simulink model "AccelPdl"  (R2023a)
settings: Solver=ode3  StartTime=0.0  StopTime=33  FixedStep=0.001  RelTol=1e-3
values from neighbouring files (symbols this model uses):
  TqCmdEPA_Forward_Final = 434.3391262014984 436.91867797860527 439.498229755712 442.07778153281885 444.65733330992566 447.42381495044009 450.91373414617271 454.40365334190523 457.89357253763791 461.38349173337048 463.56484227432378 463.86833033972778 464.17181840513183 464.47530647053583 464.77879453593988 464.89533286466883 464.89533286466883 464.89533286466883 464.89533286466883 464.89533286466883 464.64606655078757 464.    [BeginnerDevModel_Dictionary.sldd]    (also in EPATorqueOutputs.mat = [434.339126201 436.918677979 439.498229756 442.077781533 444; TqCommandGenerator.m = transpose(TqCmd_Array_Reshaped))
  TqCmdEPA_Reverse_Final = -124.07811446556342 -124.07811446556342 -124.07811446556342 -124.07811446556342 -124.0781144658778 -124.07811447343717 -124.07811448099652 -124.07811448855587 -124.07811449548642 -124.07811449548642 -124.07811449548642 -124.07811449548642 -124.07811449548642 -124.07811449548642 -124.07811449548642 -124.07001588912377 -124.01236684976388 -123.95471781040399 -123.89706877104413 -123.83941973168425 -    [BeginnerDevModel_Dictionary.sldd]    (also in EPATorqueOutputs.mat = [-124.078114466 -124.078114466 -124.078114466 -124.078114466; TqCommandGenerator.m = transpose(TqCmd_Array_Reshaped))
settings Model: DataDictionary=BeginnerDevModel_Dictionary.sldd  Creator=edward9  LastModifiedBy=edward9

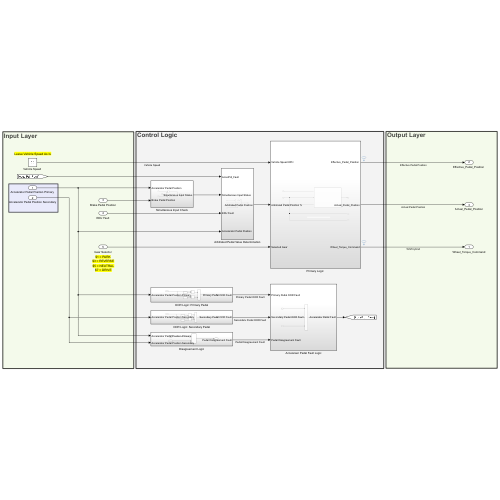
[thumbnail: Simulink's stored preview of the top-level diagram]
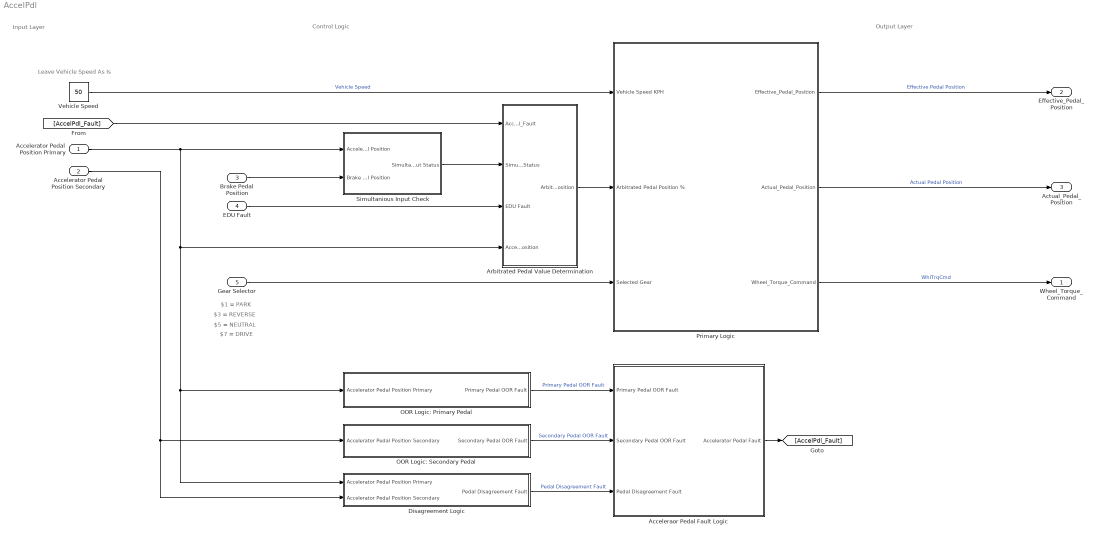
== system AccelPdl ==
  note: $7 = DRIVE
  note: $5 = NEUTRAL
  note: $3 = REVERSE
  note: Control Logic
  note: Input Layer
  note: Output Layer
  note: $1 = PARK
  note: Leave Vehicle Speed As Is
  "Accelerator Pedal Position Primary " : Inport  OutDataTypeStr=double
  Accelerator Pedal Position Secondary : Inport  Port=2  OutDataTypeStr=double
  Brake Pedal Position : Inport  Port=3  OutDataTypeStr=double
  EDU Fault : Inport  Port=4
  Gear Selector : Inport  Port=5  OutDataTypeStr=double
  Acceleraor Pedal Fault Logic : Subsystem
  Arbitrated Pedal Value Determination : Subsystem
  Disagreement Logic : Subsystem
  OOR Logic: Primary Pedal : Subsystem
  OOR Logic: Secondary Pedal : Subsystem
  "Primary Logic " : Subsystem
  Simultanious Input Check : Subsystem
  "Vehicle Speed " : Constant  Value=50
  Wheel_Torque_Command : Outport
  "Effective_Pedal_Position " : Outport  Port=2
  Actual_Pedal_Position : Outport  Port=3
  wires:
  Acceleraor Pedal Fault Logic/1(Accelerator Pedal Fault) -> [AccelPdl_Fault]
  "Vehicle Speed "/1 -> "Primary Logic "/1(Vehicle Speed KPH)  "Vehicle Speed"
  "Primary Logic "/1("Effective_Pedal_Position ") -> "Effective_Pedal_Position "/1  "Effective Pedal Position"
  "Primary Logic "/2(Actual_Pedal_Position) -> Actual_Pedal_Position/1  "Actual Pedal Position"
  Gear Selector/1 -> "Primary Logic "/3(Selected Gear)
  Arbitrated Pedal Value Determination/1(Arbitrated Pedal Position) -> "Primary Logic "/2("Arbitrated Pedal Position % ")
  "Primary Logic "/3(Wheel_Torque_Command) -> Wheel_Torque_Command/1  "WhlTrqCmd"
  Brake Pedal Position/1 -> Simultanious Input Check/2(Brake Pedal Position)
  [AccelPdl_Fault] -> Arbitrated Pedal Value Determination/1(AccelPdl_Fault)
  Simultanious Input Check/1(Simultanious Input Status) -> Arbitrated Pedal Value Determination/2(Simultanious Input Status)
  EDU Fault/1 -> Arbitrated Pedal Value Determination/3(EDU Fault)
  OOR Logic: Secondary Pedal/1(Secondary Pedal OOR Fault) -> Acceleraor Pedal Fault Logic/2(Secondary Pedal OOR Fault)  "Secondary Pedal OOR Fault"
  Disagreement Logic/1(Pedal Disagreement Fault) -> Acceleraor Pedal Fault Logic/3(Pedal Disagreement Fault)  "Pedal Disagreement Fault"
  OOR Logic: Primary Pedal/1(Primary Pedal OOR Fault) -> Acceleraor Pedal Fault Logic/1(Primary Pedal OOR Fault)  "Primary Pedal OOR Fault"
  "Accelerator Pedal Position Primary "/1 -> Simultanious Input Check/1("Accelerator Pedal Position "), Disagreement Logic/1(Accelerator Pedal Position Primary), OOR Logic: Primary Pedal/1(Accelerator Pedal Position Primary), Arbitrated Pedal Value Determination/4(Accelerator Pedal Position)
  Accelerator Pedal Position Secondary/1 -> Disagreement Logic/2(Accelerator Pedal Position Secondary), OOR Logic: Secondary Pedal/1(Accelerator Pedal Position Secondary)

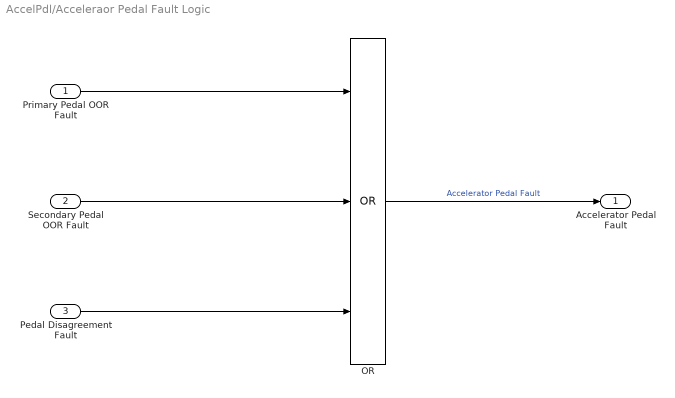
== system AccelPdl/Acceleraor Pedal Fault Logic ==
  Primary Pedal OOR Fault : Inport
  Secondary Pedal OOR Fault : Inport  Port=2
  Pedal Disagreement Fault : Inport  Port=3
  OR : Logic  Operator=OR  Inputs=3  AllPortsSameDT=off  OutDataTypeStr=boolean
  Accelerator Pedal Fault : Outport
  wires:
  Pedal Disagreement Fault/1 -> OR/3
  Secondary Pedal OOR Fault/1 -> OR/2
  Primary Pedal OOR Fault/1 -> OR/1
  OR/1 -> Accelerator Pedal Fault/1  "Accelerator Pedal Fault"

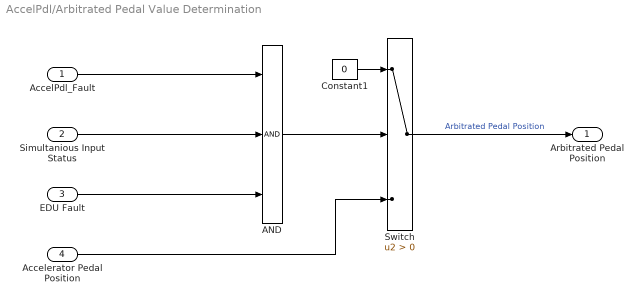
== system AccelPdl/Arbitrated Pedal Value Determination ==
  AccelPdl_Fault : Inport
  Simultanious Input Status : Inport  Port=2
  EDU Fault : Inport  Port=3
  Accelerator Pedal Position : Inport  Port=4
  AND : Logic  Inputs=3  AllPortsSameDT=off  OutDataTypeStr=boolean
  Constant1 : Constant  Value=0
  Switch : Switch  Criteria=u2 > Threshold  SaturateOnIntegerOverflow=off  InputSameDT=off
  Arbitrated Pedal Position : Outport
  wires:
  AccelPdl_Fault/1 -> AND/1
  Accelerator Pedal Position/1 -> Switch/3
  Simultanious Input Status/1 -> AND/2
  AND/1 -> Switch/2
  EDU Fault/1 -> AND/3
  Constant1/1 -> Switch/1
  Switch/1 -> Arbitrated Pedal Position/1  "Arbitrated Pedal Position"

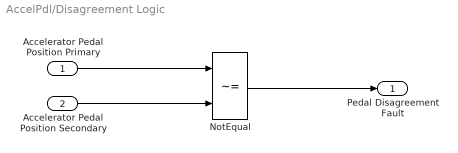
== system AccelPdl/Disagreement Logic ==
  Accelerator Pedal Position Primary : Inport
  Accelerator Pedal Position Secondary : Inport  Port=2
  NotEqual : RelationalOperator  Operator=~=  OutDataTypeStr=boolean  RndMeth=Simplest  InputSameDT=off
  Pedal Disagreement Fault : Outport
  wires:
  NotEqual/1 -> Pedal Disagreement Fault/1
  Accelerator Pedal Position Primary/1 -> NotEqual/1
  Accelerator Pedal Position Secondary/1 -> NotEqual/2

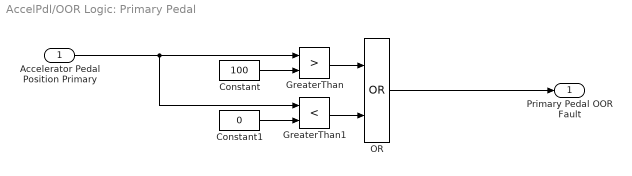
== system AccelPdl/OOR Logic: Primary Pedal ==
  Accelerator Pedal Position Primary : Inport
  Constant : Constant  Value=100
  Constant1 : Constant  Value=0
  GreaterThan : RelationalOperator  Operator=>  OutDataTypeStr=boolean  RndMeth=Simplest  InputSameDT=off
  GreaterThan1 : RelationalOperator  Operator=<  OutDataTypeStr=boolean  RndMeth=Simplest  InputSameDT=off
  OR : Logic  Operator=OR  AllPortsSameDT=off  OutDataTypeStr=boolean
  Primary Pedal OOR Fault : Outport
  wires:
  OR/1 -> Primary Pedal OOR Fault/1
  Constant1/1 -> GreaterThan1/2
  GreaterThan/1 -> OR/1
  GreaterThan1/1 -> OR/2
  Constant/1 -> GreaterThan/2
  Accelerator Pedal Position Primary/1 -> GreaterThan1/1, GreaterThan/1

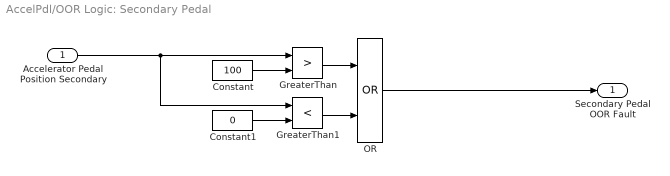
== system AccelPdl/OOR Logic: Secondary Pedal ==
  Accelerator Pedal Position Secondary : Inport
  Constant : Constant  Value=100
  Constant1 : Constant  Value=0
  GreaterThan : RelationalOperator  Operator=>  OutDataTypeStr=boolean  RndMeth=Simplest  InputSameDT=off
  GreaterThan1 : RelationalOperator  Operator=<  OutDataTypeStr=boolean  RndMeth=Simplest  InputSameDT=off
  OR : Logic  Operator=OR  AllPortsSameDT=off  OutDataTypeStr=boolean
  Secondary Pedal OOR Fault : Outport
  wires:
  OR/1 -> Secondary Pedal OOR Fault/1
  Constant1/1 -> GreaterThan1/2
  GreaterThan/1 -> OR/1
  GreaterThan1/1 -> OR/2
  Constant/1 -> GreaterThan/2
  Accelerator Pedal Position Secondary/1 -> GreaterThan1/1, GreaterThan/1

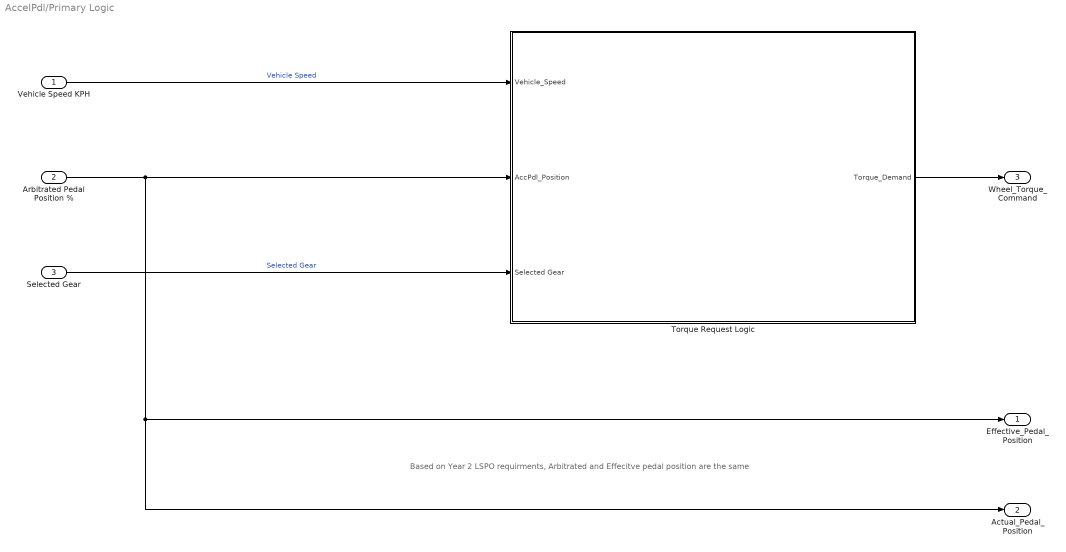
== system AccelPdl/Primary Logic  ==
  note: Based on Year 2 LSPO requirments, Arbitrated and Effecitve pedal position are the same
  Vehicle Speed KPH : Inport
  "Arbitrated Pedal Position % " : Inport  Port=2
  Selected Gear : Inport  Port=3
  Torque Request Logic : Subsystem
  "Effective_Pedal_Position " : Outport
  Actual_Pedal_Position : Outport  Port=2
  Wheel_Torque_Command : Outport  Port=3
  wires:
  Vehicle Speed KPH/1 -> Torque Request Logic/1(Vehicle_Speed)  "Vehicle Speed"
  "Arbitrated Pedal Position % "/1 -> Torque Request Logic/2(AccPdl_Position), "Effective_Pedal_Position "/1, Actual_Pedal_Position/1
  Selected Gear/1 -> Torque Request Logic/3("Selected Gear ")  "Selected Gear"
  Torque Request Logic/1("Torque_Demand ") -> Wheel_Torque_Command/1

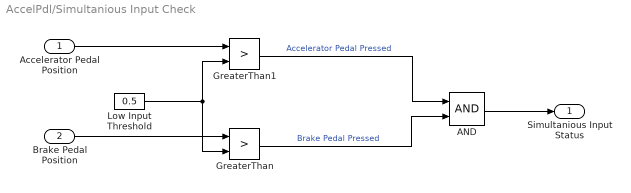
== system AccelPdl/Simultanious Input Check ==
  "Accelerator Pedal Position " : Inport
  Brake Pedal Position : Inport  Port=2
  AND : Logic  AllPortsSameDT=off  OutDataTypeStr=boolean
  GreaterThan : RelationalOperator  Operator=>  OutDataTypeStr=boolean  RndMeth=Simplest  InputSameDT=off
  GreaterThan1 : RelationalOperator  Operator=>  OutDataTypeStr=boolean  RndMeth=Simplest  InputSameDT=off
  Low Input Threshold : Constant  Value=0.5
  Simultanious Input Status : Outport
  wires:
  GreaterThan1/1 -> AND/1  "Accelerator Pedal Pressed"
  GreaterThan/1 -> AND/2  "Brake Pedal Pressed"
  Low Input Threshold/1 -> GreaterThan1/2, GreaterThan/2
  "Accelerator Pedal Position "/1 -> GreaterThan1/1
  AND/1 -> Simultanious Input Status/1
  Brake Pedal Position/1 -> GreaterThan/1

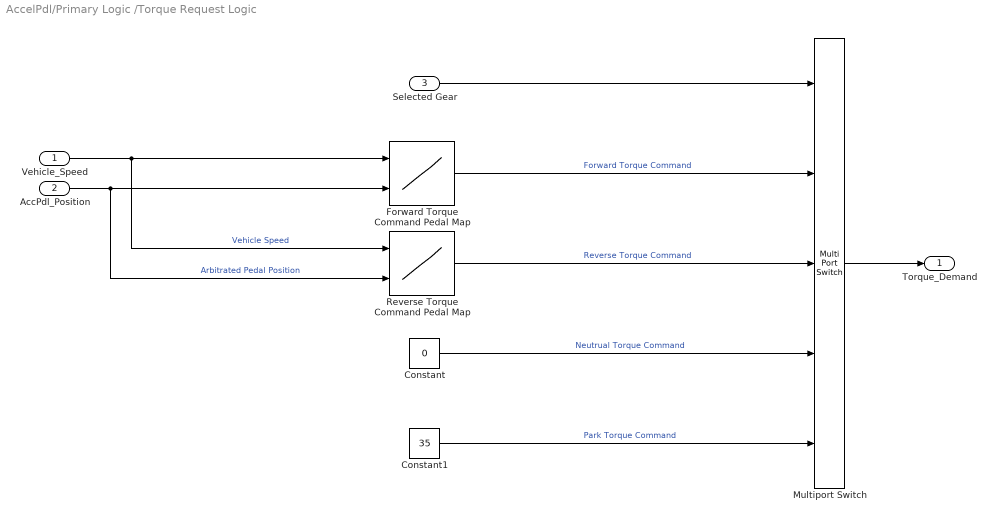
== system AccelPdl/Primary Logic /Torque Request Logic ==
  Vehicle_Speed : Inport
  AccPdl_Position : Inport  Port=2
  "Selected Gear " : Inport  Port=3
  Constant : Constant  Value=0  SampleTime=-1
  Constant1 : Constant  Value=35  SampleTime=-1
  Forward Torque Command Pedal Map : Lookup_n-D  BreakpointsForDimension1=[0:150]  BreakpointsForDimension2=[1:100]  Table=TqCmdEPA_Forward_Final*0.7  ExtrapMethod=Clip  UseLastTableValue=on  InternalRulePriority=Speed  RndMeth=Simplest
      settings: InputPortMap=u0,u1
  Multiport Switch : MultiPortSwitch  DataPortOrder=Specify indices  Inputs=4  DataPortIndices={7,3,5,1}  SaturateOnIntegerOverflow=off  InputSameDT=off
  Reverse Torque Command Pedal Map : Lookup_n-D  BreakpointsForDimension1=[0:150]  BreakpointsForDimension2=[1:100]  Table=TqCmdEPA_Reverse_Final*0.15  ExtrapMethod=Clip  UseLastTableValue=on  InternalRulePriority=Speed  RndMeth=Simplest
      settings: InputPortMap=u0,u1
  "Torque_Demand " : Outport
  wires:
  AccPdl_Position/1 -> Forward Torque Command Pedal Map/2, Reverse Torque Command Pedal Map/2  "Arbitrated Pedal Position"
  Vehicle_Speed/1 -> Forward Torque Command Pedal Map/1, Reverse Torque Command Pedal Map/1  "Vehicle Speed"
  Multiport Switch/1 -> "Torque_Demand "/1
  Forward Torque Command Pedal Map/1 -> Multiport Switch/2  "Forward Torque Command"
  Constant/1 -> Multiport Switch/4  "Neutrual Torque Command"
  "Selected Gear "/1 -> Multiport Switch/1
  Constant1/1 -> Multiport Switch/5  "Park Torque Command"
  Reverse Torque Command Pedal Map/1 -> Multiport Switch/3  "Reverse Torque Command"
